simulink model "Part_3_Simulink_With_All_Scopes_Simplified_Blocks"  (R2016a)
settings: Solver=VariableStepAuto  StartTime=0.0  StopTime=12  RelTol=1e-3
values from neighbouring files (symbols this model uses):
  Alpha = 1    [Parameters_And_Plot.m]    (also in Part5_Specified_Destinations.m)
  K12 = K(1,2)    [Parameters_And_Plot.m]    (also in Part5_Specified_Destinations.m)
  K13 = K(1,3)    [Parameters_And_Plot.m]    (also in Part5_Specified_Destinations.m)
  K14 = K(1,4)    [Parameters_And_Plot.m]    (also in Part5_Specified_Destinations.m)
  K15 = K(1,5)    [Parameters_And_Plot.m]    (also in Part5_Specified_Destinations.m)
  K21 = K(2,1)    [Parameters_And_Plot.m]    (also in Part5_Specified_Destinations.m)
  K23 = K(2,1)    [Parameters_And_Plot.m]    (also in Part5_Specified_Destinations.m)
  K24 = K(2,1)    [Parameters_And_Plot.m]    (also in Part5_Specified_Destinations.m)
  K25 = K(2,1)    [Parameters_And_Plot.m]    (also in Part5_Specified_Destinations.m)
  K31 = K(3,1)    [Parameters_And_Plot.m]    (also in Part5_Specified_Destinations.m)
  K32 = K(3,2)    [Parameters_And_Plot.m]    (also in Part5_Specified_Destinations.m)
  K34 = K(3,4)    [Parameters_And_Plot.m]    (also in Part5_Specified_Destinations.m)
  K35 = K(3,5)    [Parameters_And_Plot.m]    (also in Part5_Specified_Destinations.m)
  K41 = K(4,1)    [Parameters_And_Plot.m]    (also in Part5_Specified_Destinations.m)
  K42 = K(4,2)    [Parameters_And_Plot.m]    (also in Part5_Specified_Destinations.m)
  K43 = K(4,3)    [Parameters_And_Plot.m]    (also in Part5_Specified_Destinations.m)
  K45 = K(4,5)    [Parameters_And_Plot.m]    (also in Part5_Specified_Destinations.m)
  K51 = K(5,1)    [Parameters_And_Plot.m]    (also in Part5_Specified_Destinations.m)
  K52 = K(5,2)    [Parameters_And_Plot.m]    (also in Part5_Specified_Destinations.m)
  K53 = K(5,3)    [Parameters_And_Plot.m]    (also in Part5_Specified_Destinations.m)
  K54 = K(5,4)    [Parameters_And_Plot.m]    (also in Part5_Specified_Destinations.m)
  L = 1    [Parameters_And_Plot.m]    (also in Part5_Specified_Destinations.m)
  x1_0 = r1_0(1)    [Parameters_And_Plot.m]    (also in Part5_Specified_Destinations.m)
  x1d = r1d(1)    [Parameters_And_Plot.m]    (also in Part5_Specified_Destinations.m)
  x2_0 = r2_0(1)    [Parameters_And_Plot.m]    (also in Part5_Specified_Destinations.m)
  x2d = r2d(1)    [Parameters_And_Plot.m]    (also in Part5_Specified_Destinations.m)
  x3_0 = r3_0(1)    [Parameters_And_Plot.m]    (also in Part5_Specified_Destinations.m)
  x3d = r3d(1)    [Parameters_And_Plot.m]    (also in Part5_Specified_Destinations.m)
  x4_0 = r4_0(1)    [Parameters_And_Plot.m]    (also in Part5_Specified_Destinations.m)
  x4d = r4d(1)    [Parameters_And_Plot.m]    (also in Part5_Specified_Destinations.m)
  x5_0 = r5_0(1)    [Parameters_And_Plot.m]    (also in Part5_Specified_Destinations.m)
  x5d = r5d(1)    [Parameters_And_Plot.m]    (also in Part5_Specified_Destinations.m)
  y1_0 = r1_0(2)    [Parameters_And_Plot.m]    (also in Part5_Specified_Destinations.m)
  y1d = r1d(2)    [Parameters_And_Plot.m]    (also in Part5_Specified_Destinations.m)
  y2_0 = r2_0(2)    [Parameters_And_Plot.m]    (also in Part5_Specified_Destinations.m)
  y2d = r2d(2)    [Parameters_And_Plot.m]    (also in Part5_Specified_Destinations.m)
  y3_0 = r3_0(2)    [Parameters_And_Plot.m]    (also in Part5_Specified_Destinations.m)
  y3d = r3d(2)    [Parameters_And_Plot.m]    (also in Part5_Specified_Destinations.m)
  y4_0 = r4_0(2)    [Parameters_And_Plot.m]    (also in Part5_Specified_Destinations.m)
  y4d = r4d(2)    [Parameters_And_Plot.m]    (also in Part5_Specified_Destinations.m)
  y5_0 = r5_0(2)    [Parameters_And_Plot.m]    (also in Part5_Specified_Destinations.m)
  y5d = r5d(2)    [Parameters_And_Plot.m]    (also in Part5_Specified_Destinations.m)
settings Model: Creator=Mohammad Hammoud  LastModifiedBy=Mohammad Hammoud

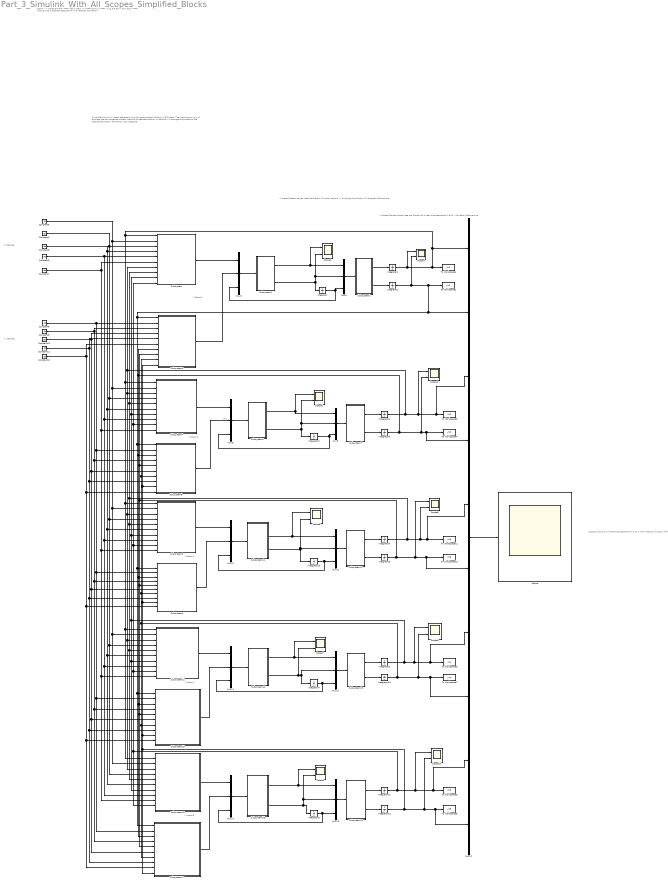
== system Part_3_Simulink_With_All_Scopes_Simplified_Blocks ==
  note: < Robot 1
  note: Yi desired
  note: Xi desired
  note: Scope to show all Linear Displacements
      | Xi and Yi of All Robots, function of Time
  note: In these Scopes we can see the Graphs of Linear
      | displacements Xi and Yi for each Robot alone
  note: In these Scopes we can see the Graphs of Linear Velocity Vi and Angular Velocity Wi for each Robot alone
  note: Part 3: " I mplement the controlled system in Matlab/Simulink "
      | Driving 5 Robots from their Initial Positions to a Desired destination
      | (with Desired Formation)
  note: Simplified Simulink Model representing a Consensus-based Control of 5 Robots,
      | The used control Law Ui, ensures the convergence of each robot to its desired position
      | In addition, it arranges the shape of the Desired Formation (Formation Convergence)
  note: Uy2
  note: < Robot 2
  note: < Robot 3
  note: < Robot 4
  note: < Robot 5
  Constant10 : Constant  Value=y3d
  Constant11 : Constant  Value=y4d
  Constant12 : Constant  Value=y5d
  Constant3 : Constant  Value=x1d
  Constant4 : Constant  Value=x2d
  Constant5 : Constant  Value=x3d
  Constant6 : Constant  Value=x4d
  Constant7 : Constant  Value=x5d
  Constant8 : Constant  Value=y1d
  Constant9 : Constant  Value=y2d
  Integrator{,1,4,6,10} (5 alike) : Integrator
  "Integrator1 " : Integrator  InitialCondition=x1_0
  "Integrator10 " : Integrator  InitialCondition=y4_0
  "Integrator11 " : Integrator  InitialCondition=x5_0
  "Integrator12 " : Integrator  InitialCondition=y5_0
  Integrator2 : Integrator  InitialCondition=y1_0
  Integrator3 : Integrator  InitialCondition=y2_0
  "Integrator4 " : Integrator  InitialCondition=x2_0
  "Integrator5 " : Integrator  InitialCondition=x3_0
  "Integrator8 " : Integrator  InitialCondition=y3_0
  "Integrator9 " : Integrator  InitialCondition=x4_0
  Mux{5..6,8..9,11..12,14..15,21..22} (10 alike) : Mux  Inputs=3
  Mux17 : Mux  Inputs=10
  Scope : Scope
  Scope{1..10} (10 alike) : Scope  NumInputPorts=2
  Subsystem : Subsystem
  Subsystem1 : Subsystem
  Subsystem10 : Subsystem
  Subsystem11 : Subsystem
  Subsystem12 : Subsystem
  Subsystem13 : Subsystem
  Subsystem14 : Subsystem
  Subsystem15 : Subsystem
  Subsystem16 : Subsystem
  Subsystem17 : Subsystem
  Subsystem18 : Subsystem
  Subsystem19 : Subsystem
  Subsystem2 : Subsystem
  Subsystem3 : Subsystem
  Subsystem4 : Subsystem
  Subsystem5 : Subsystem
  Subsystem6 : Subsystem
  Subsystem7 : Subsystem
  Subsystem8 : Subsystem
  Subsystem9 : Subsystem
  To Workspace1 : ToWorkspace  VariableName=xh1  SampleTime=-1
  To Workspace11 : ToWorkspace  VariableName=xh3  SampleTime=-1
  To Workspace12 : ToWorkspace  VariableName=yh3  SampleTime=-1
  To Workspace2 : ToWorkspace  VariableName=yh1  SampleTime=-1
  To Workspace3 : ToWorkspace  VariableName=xh2  SampleTime=-1
  To Workspace4 : ToWorkspace  VariableName=yh2  SampleTime=-1
  To Workspace5 : ToWorkspace  VariableName=xh5  SampleTime=-1
  To Workspace6 : ToWorkspace  VariableName=xh4  SampleTime=-1
  To Workspace7 : ToWorkspace  VariableName=yh4  SampleTime=-1
  To Workspace8 : ToWorkspace  VariableName=yh5  SampleTime=-1
  wires:
  Constant3/1 -> Subsystem16/2(In2), Subsystem12/2(In2), Subsystem8/2(In2), Subsystem4/2(In2), Subsystem/2(In2)  "x1d"
  Constant4/1 -> Subsystem16/4(In4), Subsystem12/4(In4), Subsystem8/4(In4), Subsystem4/4(In4), Subsystem/3(In3)  "x2d"
  Constant5/1 -> Subsystem16/6(In6), Subsystem12/6(In6), Subsystem8/6(In6), Subsystem4/6(In6), Subsystem/4(In4)  "x3d"
  Constant6/1 -> Subsystem16/8(In8), Subsystem12/8(In8), Subsystem8/8(In8), Subsystem4/8(In8), Subsystem/5(In5)  "x4d"
  Constant7/1 -> Subsystem16/9(In9), Subsystem12/10(In10), Subsystem8/10(In10), Subsystem4/10(In10), Subsystem/6(In6)  "x5d"
  Constant8/1 -> Subsystem17/2(In2), Subsystem13/2(In2), Subsystem9/2(In2), Subsystem5/2(In2), Subsystem3/2(In2)  "y1d"
  Constant9/1 -> Subsystem17/4(In4), Subsystem13/4(In4), Subsystem9/4(In4), Subsystem5/4(In4), Subsystem3/3(In3)  "y2d"
  Constant10/1 -> Subsystem3/4(In4), Subsystem17/6(In6), Subsystem13/6(In6), Subsystem9/6(In6), Subsystem5/6(In6)  "y3d"
  Constant11/1 -> Subsystem3/5(In5), Subsystem17/8(In8), Subsystem13/8(In8), Subsystem9/8(In8), Subsystem5/8(In8)  "y4d"
  Constant12/1 -> Subsystem3/6(In6), Subsystem17/9(In9), Subsystem13/10(In10), Subsystem9/10(In10), Subsystem5/10(In10)  "y5d"
  Integrator/1 -> Mux6/3, Mux5/3  "Theta 1"
  "Integrator1 "/1 -> Scope4/1, Subsystem/1(In1), Subsystem16/1(In1), Subsystem12/1(In1), Subsystem8/1(In1), Subsystem4/1(In1), Mux17/1, To Workspace1/1  "x1"
  Integrator2/1 -> To Workspace2/1, Subsystem3/1(In1), Subsystem17/1(In1), Subsystem13/1(In1), Subsystem9/1(In1), Subsystem5/1(In1), Mux17/2, Scope4/2  "y1"
  Integrator1/1 -> Mux8/3, Mux9/3  "Theta 2"
  "Integrator4 "/1 -> Subsystem/7(In7), Subsystem16/3(In3), Subsystem12/3(In3), Subsystem8/3(In3), Subsystem4/3(In3), Scope3/1, Mux17/3, To Workspace3/1  "x2"
  Integrator3/1 -> Subsystem3/7(In7), Subsystem5/3(In3), Subsystem13/3(In3), Subsystem17/3(In3), Subsystem9/3(In3), Scope3/2, To Workspace4/1, Mux17/4  "y2"
  Integrator10/1 -> Mux22/3, Mux21/3  "Theta 3"
  "Integrator5 "/1 -> Subsystem/8(In8), Subsystem4/5(In5), Subsystem16/5(In5), Subsystem12/5(In5), Subsystem8/5(In5), Scope6/2, Mux17/5, To Workspace11/1  "x3"
  "Integrator8 "/1 -> Subsystem3/8(In8), Subsystem5/5(In5), Subsystem17/5(In5), Subsystem13/5(In5), Subsystem9/5(In5), Scope6/1, To Workspace12/1, Mux17/6  "y3"
  Integrator4/1 -> Mux11/3, Mux12/3  "Theta 4"
  "Integrator9 "/1 -> To Workspace6/1, Mux17/7, Scope8/1, Subsystem16/7(In7), Subsystem12/7(In7), Subsystem/9(In9), Subsystem4/7(In7), Subsystem8/7(In7)  "x4"
  "Integrator10 "/1 -> To Workspace7/1, Mux17/8, Scope8/2, Subsystem3/9(In9), Subsystem5/7(In7), Subsystem9/7(In7), Subsystem17/7(In7), Subsystem13/7(In7)  "y4"
  Integrator6/1 -> Mux15/3, Mux14/3  "Theta 5"
  "Integrator11 "/1 -> To Workspace5/1, Mux17/9, Scope10/1, Subsystem/10(In10), Subsystem4/9(In9), Subsystem8/9(In9), Subsystem12/9(In9), Subsystem16/10(In10)  "x5"
  "Integrator12 "/1 -> To Workspace8/1, Mux17/10, Scope10/2, Subsystem17/10(In10), Subsystem3/10(In10), Subsystem5/9(In9), Subsystem9/9(In9), Subsystem13/9(In9)  "y5"
  Mux17/1 -> Scope/1
  Subsystem/1(Out1) -> Mux5/1  "Ux1"
  Subsystem1/2(Out2) -> Scope1/2, Mux6/2, Integrator/1  "W1"
  Subsystem1/1(Out1) -> Scope1/1, Mux6/1  "V1"
  Mux5/1 -> Subsystem1/1(In1)
  Mux6/1 -> Subsystem2/1(In1)
  Subsystem2/1(Out1) -> "Integrator1 "/1  "x1dot"
  Subsystem2/2(Out2) -> Integrator2/1  "y1dot"
  Subsystem3/1(Out1) -> Mux5/2  "Uy1"
  Subsystem4/1(Out1) -> Mux8/1  "Ux2"
  Subsystem5/1(Out1) -> Mux8/2
  Subsystem6/2(Out2) -> Integrator1/1, Scope2/2, Mux9/2  "W2"
  Subsystem6/1(Out1) -> Mux9/1, Scope2/1  "V2"
  Mux8/1 -> Subsystem6/1(In1)
  Mux9/1 -> Subsystem7/1(In1)
  Subsystem7/1(Out1) -> "Integrator4 "/1  "x2dot"
  Subsystem7/2(Out2) -> Integrator3/1  "y2dot"
  Subsystem8/1(Out1) -> Mux21/1  "Ux3"
  Subsystem9/1(Out1) -> Mux21/2  "Uy3"
  Subsystem10/1(Out1) -> Scope5/1, Mux22/1  "V3"
  Subsystem10/2(Out2) -> Integrator10/1, Scope5/2, Mux22/2  "W3"
  Mux21/1 -> Subsystem10/1(In1)
  Mux22/1 -> Subsystem11/1(In1)
  Subsystem11/1(Out1) -> "Integrator5 "/1  "x3dot"
  Subsystem11/2(Out2) -> "Integrator8 "/1  "y3dot"
  Subsystem12/1(Out1) -> Mux11/1  "Ux4"
  Subsystem13/1(Out1) -> Mux11/2  "Uy4"
  Subsystem14/1(Out1) -> Scope7/1, Mux12/1  "V4"
  Subsystem14/2(Out2) -> Scope7/2, Mux12/2, Integrator4/1  "W4"
  Mux11/1 -> Subsystem14/1(In1)
  Mux12/1 -> Subsystem15/1(In1)
  Subsystem15/1(Out1) -> "Integrator9 "/1  "x4dot"
  Subsystem15/2(Out2) -> "Integrator10 "/1  "y4dot"
  Subsystem16/1(Out1) -> Mux14/1  "Ux5"
  Subsystem17/1(Out1) -> Mux14/2  "Uy5"
  Subsystem18/1(Out1) -> Scope9/1, Mux15/1  "V5"
  Subsystem18/2(Out2) -> Integrator6/1, Scope9/2, Mux15/2  "W5"
  Mux14/1 -> Subsystem18/1(In1)
  Mux15/1 -> Subsystem19/1(In1)
  Subsystem19/1(Out1) -> "Integrator11 "/1  "x5dot"
  Subsystem19/2(Out2) -> "Integrator12 "/1  "y5dot"

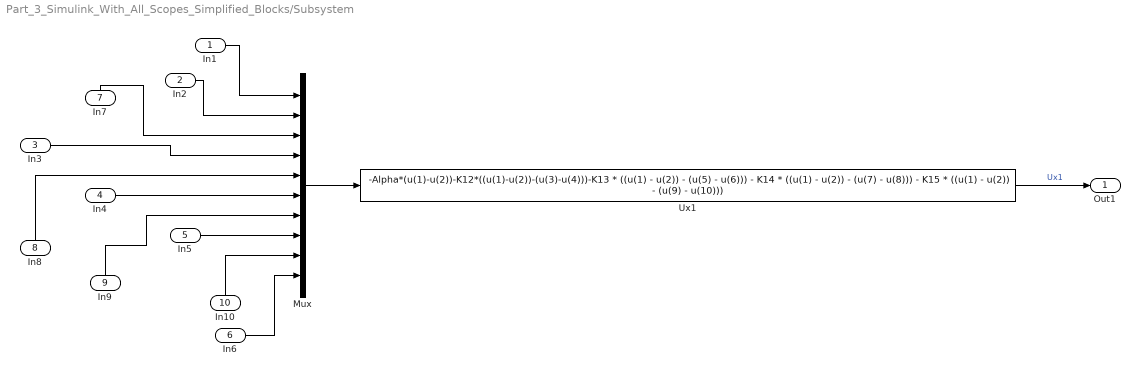
== system Part_3_Simulink_With_All_Scopes_Simplified_Blocks/Subsystem ==
  In1 : Inport
  In2 : Inport  Port=2
  In3 : Inport  Port=3
  In4 : Inport  Port=4
  In5 : Inport  Port=5
  In6 : Inport  Port=6
  In7 : Inport  Port=7
  In8 : Inport  Port=8
  In9 : Inport  Port=9
  In10 : Inport  Port=10
  Mux : Mux  Inputs=10
  Ux1 : Fcn  Expr=-Alpha*(u(1)-u(2))-K12*((u(1)-u(2))-(u(3)-u(4)))-K13 * ((u(1) - u(2)) - (u(5) - u(6))) - K14 * ((u(1) - u(2)) - (u(7) - u(8))) - K15 * ((u(1) - u(2)) - (u(9) - u(10)))
  Out1 : Outport
  wires:
  In9/1 -> Mux/7
  In2/1 -> Mux/2
  In3/1 -> Mux/4
  In4/1 -> Mux/6
  In1/1 -> Mux/1
  In6/1 -> Mux/10
  In5/1 -> Mux/8
  In10/1 -> Mux/9
  In8/1 -> Mux/5
  In7/1 -> Mux/3
  Mux/1 -> Ux1/1
  Ux1/1 -> Out1/1  "Ux1"

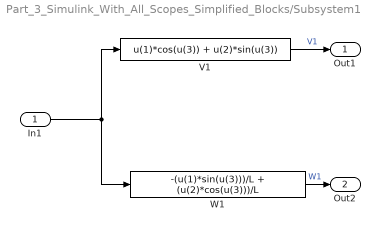
== system Part_3_Simulink_With_All_Scopes_Simplified_Blocks/Subsystem1 ==
  In1 : Inport
  V1 : Fcn  Expr=u(1)*cos(u(3)) + u(2)*sin(u(3))
  W1 : Fcn  Expr=-(u(1)*sin(u(3)))/L + (u(2)*cos(u(3)))/L
  Out1 : Outport
  Out2 : Outport  Port=2
  wires:
  In1/1 -> V1/1, W1/1
  V1/1 -> Out1/1  "V1"
  W1/1 -> Out2/1  "W1"

== system Part_3_Simulink_With_All_Scopes_Simplified_Blocks/Subsystem10 ==
  In1 : Inport
  V3 : Fcn  Expr=u(1)*cos(u(3)) + u(2)*sin(u(3))
  W3 : Fcn  Expr=-(u(1)*sin(u(3)))/L + (u(2)*cos(u(3)))/L
  Out1 : Outport
  Out2 : Outport  Port=2
  wires:
  W3/1 -> Out2/1  "W3"
  V3/1 -> Out1/1  "V3"
  In1/1 -> V3/1, W3/1

== system Part_3_Simulink_With_All_Scopes_Simplified_Blocks/Subsystem11 ==
  In1 : Inport
  Xhdot 3 : Fcn  Expr=u(1)*cos(u(3)) - L*u(2)*sin(u(3))
  Yhdot 3 : Fcn  Expr=u(1)*sin(u(3)) + L*u(2)*cos(u(3))
  Out1 : Outport
  Out2 : Outport  Port=2
  wires:
  In1/1 -> Yhdot 3/1, Xhdot 3/1
  Yhdot 3/1 -> Out2/1
  Xhdot 3/1 -> Out1/1

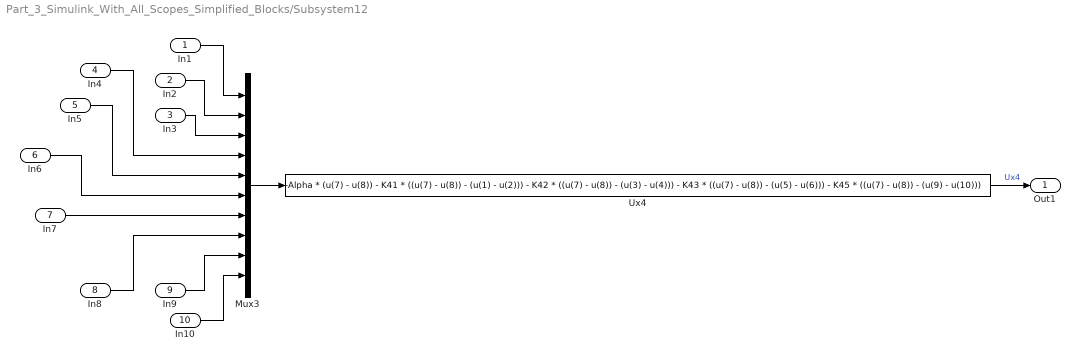
== system Part_3_Simulink_With_All_Scopes_Simplified_Blocks/Subsystem12 ==
  In1 : Inport
  In2 : Inport  Port=2
  In3 : Inport  Port=3
  In4 : Inport  Port=4
  In5 : Inport  Port=5
  In6 : Inport  Port=6
  In7 : Inport  Port=7
  In8 : Inport  Port=8
  In9 : Inport  Port=9
  In10 : Inport  Port=10
  Mux3 : Mux  Inputs=10
  Ux4 : Fcn  Expr=-Alpha * (u(7) - u(8)) - K41 * ((u(7) - u(8)) - (u(1) - u(2))) - K42 * ((u(7) - u(8)) - (u(3) - u(4))) - K43 * ((u(7) - u(8)) - (u(5) - u(6))) - K45 * ((u(7) - u(8)) - (u(9) - u(10)))
  Out1 : Outport
  wires:
  In9/1 -> Mux3/9
  In3/1 -> Mux3/3
  In7/1 -> Mux3/7
  In4/1 -> Mux3/4
  In10/1 -> Mux3/10
  In1/1 -> Mux3/1
  In2/1 -> Mux3/2
  In5/1 -> Mux3/5
  In6/1 -> Mux3/6
  In8/1 -> Mux3/8
  Mux3/1 -> Ux4/1
  Ux4/1 -> Out1/1  "Ux4"

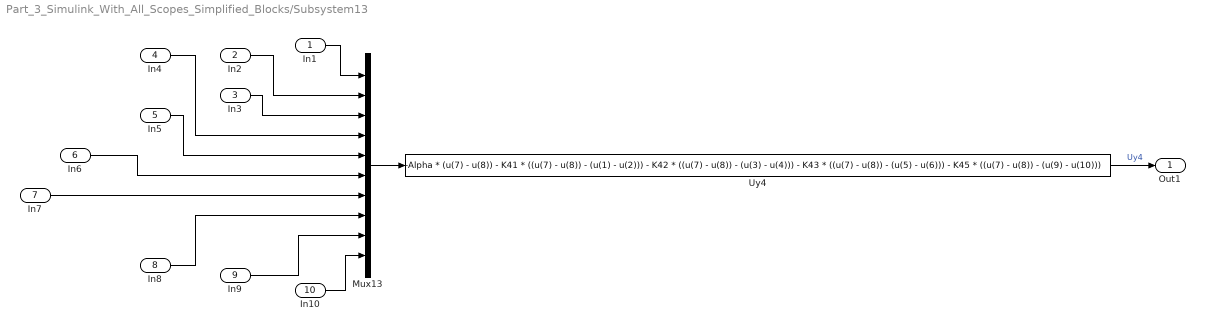
== system Part_3_Simulink_With_All_Scopes_Simplified_Blocks/Subsystem13 ==
  In1 : Inport
  In2 : Inport  Port=2
  In3 : Inport  Port=3
  In4 : Inport  Port=4
  In5 : Inport  Port=5
  In6 : Inport  Port=6
  In7 : Inport  Port=7
  In8 : Inport  Port=8
  In9 : Inport  Port=9
  In10 : Inport  Port=10
  Mux13 : Mux  Inputs=10
  Uy4 : Fcn  Expr=-Alpha * (u(7) - u(8)) - K41 * ((u(7) - u(8)) - (u(1) - u(2))) - K42 * ((u(7) - u(8)) - (u(3) - u(4))) - K43 * ((u(7) - u(8)) - (u(5) - u(6))) - K45 * ((u(7) - u(8)) - (u(9) - u(10)))
  Out1 : Outport
  wires:
  In5/1 -> Mux13/5
  In1/1 -> Mux13/1
  In7/1 -> Mux13/7
  In6/1 -> Mux13/6
  In9/1 -> Mux13/9
  In4/1 -> Mux13/4
  In8/1 -> Mux13/8
  In2/1 -> Mux13/2
  In10/1 -> Mux13/10
  In3/1 -> Mux13/3
  Mux13/1 -> Uy4/1
  Uy4/1 -> Out1/1  "Uy4"

== system Part_3_Simulink_With_All_Scopes_Simplified_Blocks/Subsystem14 ==
  In1 : Inport
  V4 : Fcn  Expr=u(1)*cos(u(3)) + u(2)*sin(u(3))
  W4 : Fcn  Expr=-(u(1)*sin(u(3)))/L + (u(2)*cos(u(3)))/L
  Out1 : Outport
  Out2 : Outport  Port=2
  wires:
  In1/1 -> W4/1, V4/1
  W4/1 -> Out2/1  "W4"
  V4/1 -> Out1/1  "V4"

== system Part_3_Simulink_With_All_Scopes_Simplified_Blocks/Subsystem15 ==
  In1 : Inport
  Xhdot 4 : Fcn  Expr=u(1)*cos(u(3)) - L*u(2)*sin(u(3))
  Yhdot 4 : Fcn  Expr=u(1)*sin(u(3)) + L*u(2)*cos(u(3))
  Out1 : Outport
  Out2 : Outport  Port=2
  wires:
  Xhdot 4/1 -> Out1/1
  In1/1 -> Yhdot 4/1, Xhdot 4/1
  Yhdot 4/1 -> Out2/1

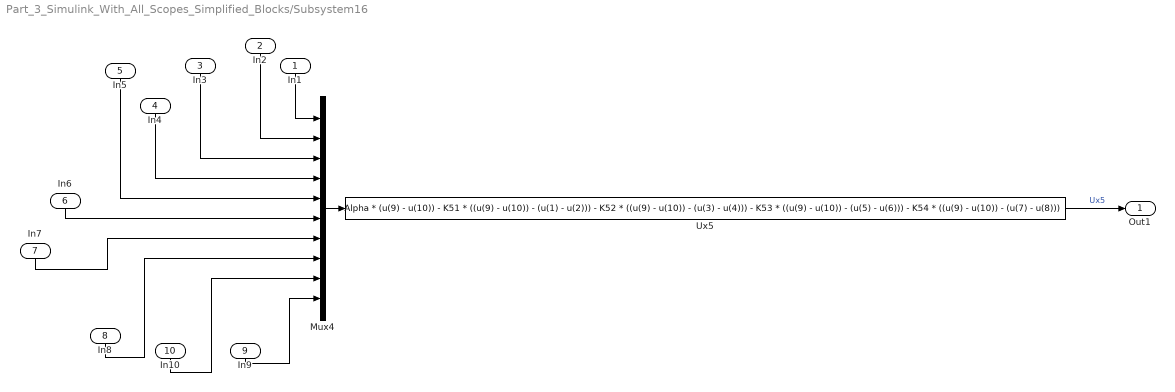
== system Part_3_Simulink_With_All_Scopes_Simplified_Blocks/Subsystem16 ==
  In1 : Inport
  In2 : Inport  Port=2
  In3 : Inport  Port=3
  In4 : Inport  Port=4
  In5 : Inport  Port=5
  In6 : Inport  Port=6
  In7 : Inport  Port=7
  In8 : Inport  Port=8
  In9 : Inport  Port=9
  In10 : Inport  Port=10
  Mux4 : Mux  Inputs=10
  Ux5 : Fcn  Expr=-Alpha * (u(9) - u(10)) - K51 * ((u(9) - u(10)) - (u(1) - u(2))) - K52 * ((u(9) - u(10)) - (u(3) - u(4))) - K53 * ((u(9) - u(10)) - (u(5) - u(6))) - K54 * ((u(9) - u(10)) - (u(7) - u(8)))
  Out1 : Outport
  wires:
  Mux4/1 -> Ux5/1
  Ux5/1 -> Out1/1  "Ux5"
  In6/1 -> Mux4/6
  In10/1 -> Mux4/9
  In9/1 -> Mux4/10
  In4/1 -> Mux4/4
  In8/1 -> Mux4/8
  In1/1 -> Mux4/1
  In2/1 -> Mux4/2
  In3/1 -> Mux4/3
  In7/1 -> Mux4/7
  In5/1 -> Mux4/5

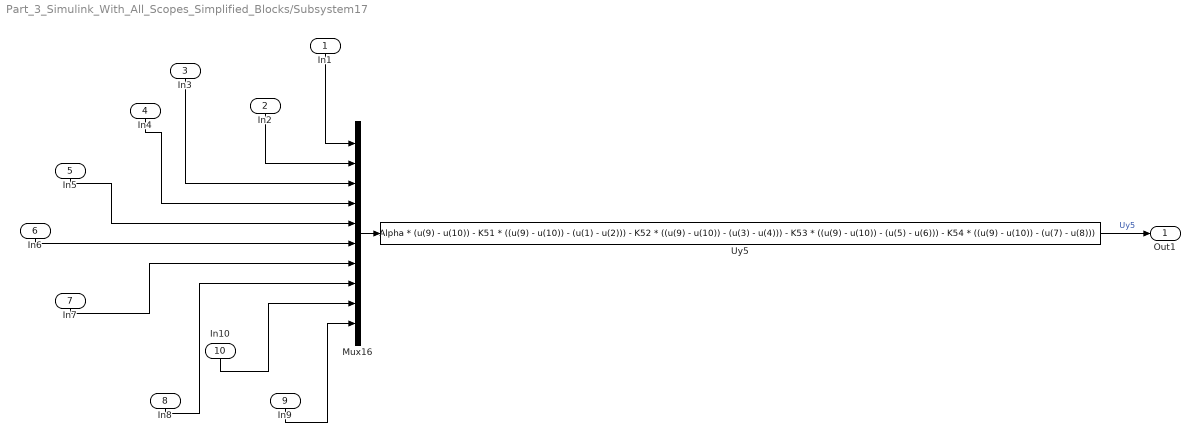
== system Part_3_Simulink_With_All_Scopes_Simplified_Blocks/Subsystem17 ==
  In1 : Inport
  In2 : Inport  Port=2
  In3 : Inport  Port=3
  In4 : Inport  Port=4
  In5 : Inport  Port=5
  In6 : Inport  Port=6
  In7 : Inport  Port=7
  In8 : Inport  Port=8
  In9 : Inport  Port=9
  In10 : Inport  Port=10
  Mux16 : Mux  Inputs=10
  Uy5 : Fcn  Expr=-Alpha * (u(9) - u(10)) - K51 * ((u(9) - u(10)) - (u(1) - u(2))) - K52 * ((u(9) - u(10)) - (u(3) - u(4))) - K53 * ((u(9) - u(10)) - (u(5) - u(6))) - K54 * ((u(9) - u(10)) - (u(7) - u(8)))
  Out1 : Outport
  wires:
  In10/1 -> Mux16/9
  In8/1 -> Mux16/8
  In4/1 -> Mux16/4
  In5/1 -> Mux16/5
  In2/1 -> Mux16/2
  In1/1 -> Mux16/1
  In6/1 -> Mux16/6
  In7/1 -> Mux16/7
  In3/1 -> Mux16/3
  In9/1 -> Mux16/10
  Mux16/1 -> Uy5/1
  Uy5/1 -> Out1/1  "Uy5"

== system Part_3_Simulink_With_All_Scopes_Simplified_Blocks/Subsystem18 ==
  In1 : Inport
  V5 : Fcn  Expr=u(1)*cos(u(3)) + u(2)*sin(u(3))
  W5 : Fcn  Expr=-(u(1)*sin(u(3)))/L + (u(2)*cos(u(3)))/L
  Out1 : Outport
  Out2 : Outport  Port=2
  wires:
  W5/1 -> Out2/1  "W5"
  In1/1 -> W5/1, V5/1
  V5/1 -> Out1/1  "V5"

== system Part_3_Simulink_With_All_Scopes_Simplified_Blocks/Subsystem19 ==
  In1 : Inport
  Xhdot 5 : Fcn  Expr=u(1)*cos(u(3)) - L*u(2)*sin(u(3))
  Yhdot 5 : Fcn  Expr=u(1)*sin(u(3)) + L*u(2)*cos(u(3))
  Out1 : Outport
  Out2 : Outport  Port=2
  wires:
  In1/1 -> Yhdot 5/1, Xhdot 5/1
  Yhdot 5/1 -> Out2/1
  Xhdot 5/1 -> Out1/1

== system Part_3_Simulink_With_All_Scopes_Simplified_Blocks/Subsystem2 ==
  In1 : Inport
  Xhdot 1 : Fcn  Expr=u(1)*cos(u(3)) - L*u(2)*sin(u(3))
  Yhdot 1 : Fcn  Expr=u(1)*sin(u(3)) + L*u(2)*cos(u(3))
  Out1 : Outport
  Out2 : Outport  Port=2
  wires:
  In1/1 -> Xhdot 1/1, Yhdot 1/1
  Yhdot 1/1 -> Out2/1
  Xhdot 1/1 -> Out1/1

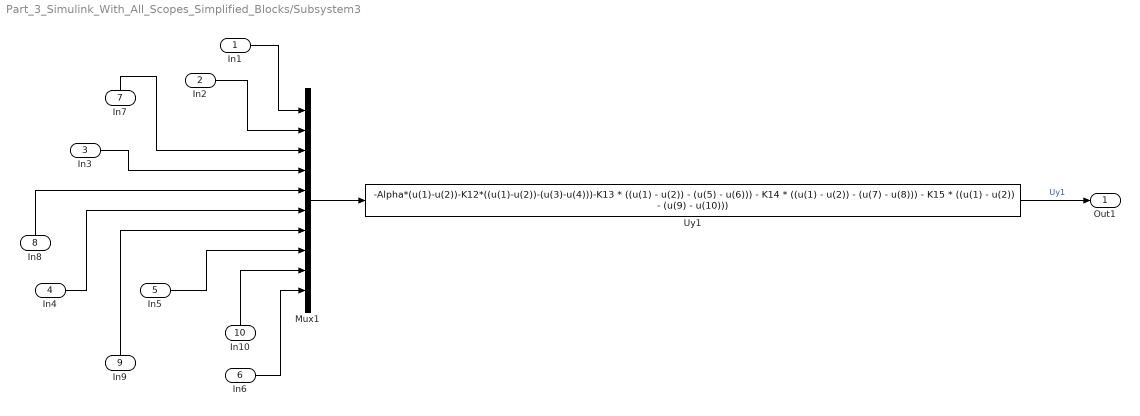
== system Part_3_Simulink_With_All_Scopes_Simplified_Blocks/Subsystem3 ==
  In1 : Inport
  In2 : Inport  Port=2
  In3 : Inport  Port=3
  In4 : Inport  Port=4
  In5 : Inport  Port=5
  In6 : Inport  Port=6
  In7 : Inport  Port=7
  In8 : Inport  Port=8
  In9 : Inport  Port=9
  In10 : Inport  Port=10
  Mux1 : Mux  Inputs=10
  Uy1 : Fcn  Expr=-Alpha*(u(1)-u(2))-K12*((u(1)-u(2))-(u(3)-u(4)))-K13 * ((u(1) - u(2)) - (u(5) - u(6))) - K14 * ((u(1) - u(2)) - (u(7) - u(8))) - K15 * ((u(1) - u(2)) - (u(9) - u(10)))
  Out1 : Outport
  wires:
  In10/1 -> Mux1/9
  In9/1 -> Mux1/7
  In8/1 -> Mux1/5
  In5/1 -> Mux1/8
  In7/1 -> Mux1/3
  In1/1 -> Mux1/1
  In3/1 -> Mux1/4
  In4/1 -> Mux1/6
  In6/1 -> Mux1/10
  In2/1 -> Mux1/2
  Mux1/1 -> Uy1/1
  Uy1/1 -> Out1/1  "Uy1"

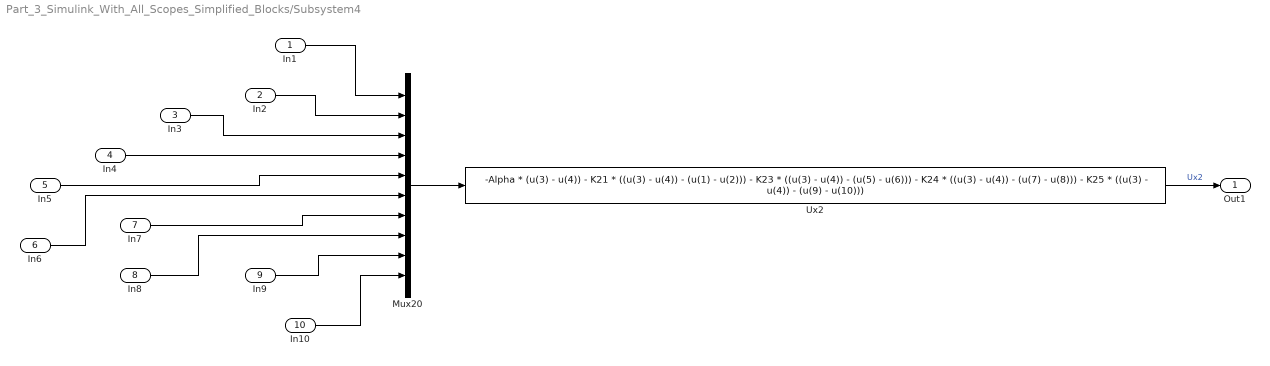
== system Part_3_Simulink_With_All_Scopes_Simplified_Blocks/Subsystem4 ==
  In1 : Inport
  In2 : Inport  Port=2
  In3 : Inport  Port=3
  In4 : Inport  Port=4
  In5 : Inport  Port=5
  In6 : Inport  Port=6
  In7 : Inport  Port=7
  In8 : Inport  Port=8
  In9 : Inport  Port=9
  In10 : Inport  Port=10
  Mux20 : Mux  Inputs=10
  Ux2 : Fcn  Expr=-Alpha * (u(3) - u(4)) - K21 * ((u(3) - u(4)) - (u(1) - u(2))) - K23 * ((u(3) - u(4)) - (u(5) - u(6))) - K24 * ((u(3) - u(4)) - (u(7) - u(8))) - K25 * ((u(3) - u(4)) - (u(9) - u(10)))
  Out1 : Outport
  wires:
  In5/1 -> Mux20/5
  In7/1 -> Mux20/7
  In8/1 -> Mux20/8
  In10/1 -> Mux20/10
  In6/1 -> Mux20/6
  In4/1 -> Mux20/4
  In1/1 -> Mux20/1
  In3/1 -> Mux20/3
  In9/1 -> Mux20/9
  In2/1 -> Mux20/2
  Mux20/1 -> Ux2/1
  Ux2/1 -> Out1/1  "Ux2"

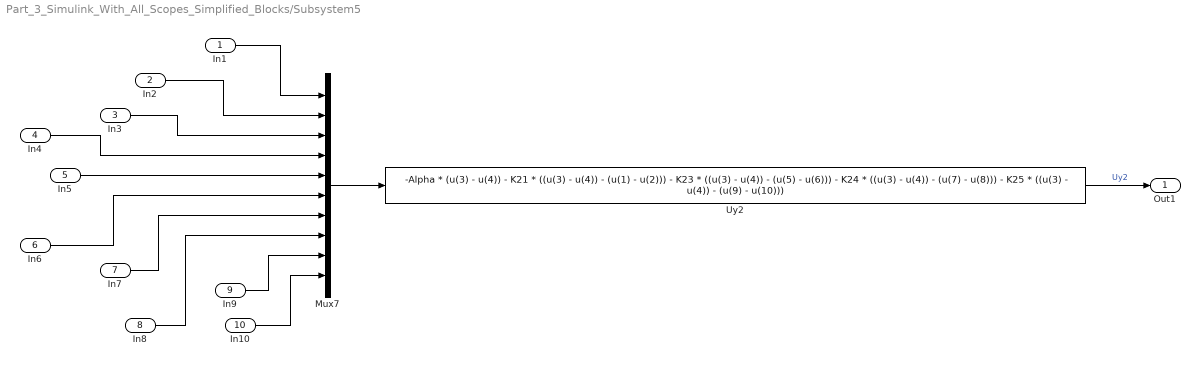
== system Part_3_Simulink_With_All_Scopes_Simplified_Blocks/Subsystem5 ==
  In1 : Inport
  In2 : Inport  Port=2
  In3 : Inport  Port=3
  In4 : Inport  Port=4
  In5 : Inport  Port=5
  In6 : Inport  Port=6
  In7 : Inport  Port=7
  In8 : Inport  Port=8
  In9 : Inport  Port=9
  In10 : Inport  Port=10
  Mux7 : Mux  Inputs=10
  Uy2 : Fcn  Expr=-Alpha * (u(3) - u(4)) - K21 * ((u(3) - u(4)) - (u(1) - u(2))) - K23 * ((u(3) - u(4)) - (u(5) - u(6))) - K24 * ((u(3) - u(4)) - (u(7) - u(8))) - K25 * ((u(3) - u(4)) - (u(9) - u(10)))
  Out1 : Outport
  wires:
  In7/1 -> Mux7/7
  In5/1 -> Mux7/5
  In6/1 -> Mux7/6
  In2/1 -> Mux7/2
  In3/1 -> Mux7/3
  In8/1 -> Mux7/8
  In9/1 -> Mux7/9
  In1/1 -> Mux7/1
  In10/1 -> Mux7/10
  In4/1 -> Mux7/4
  Mux7/1 -> Uy2/1
  Uy2/1 -> Out1/1  "Uy2"

== system Part_3_Simulink_With_All_Scopes_Simplified_Blocks/Subsystem6 ==
  In1 : Inport
  V2 : Fcn  Expr=u(1)*cos(u(3)) + u(2)*sin(u(3))
  W2 : Fcn  Expr=-(u(1)*sin(u(3)))/L + (u(2)*cos(u(3)))/L
  Out1 : Outport
  Out2 : Outport  Port=2
  wires:
  In1/1 -> W2/1, V2/1
  W2/1 -> Out2/1  "W2"
  V2/1 -> Out1/1  "V2"

== system Part_3_Simulink_With_All_Scopes_Simplified_Blocks/Subsystem7 ==
  In1 : Inport
  Xhdot 2 : Fcn  Expr=u(1)*cos(u(3)) - L*u(2)*sin(u(3))
  Yhdot 2 : Fcn  Expr=u(1)*sin(u(3)) + L*u(2)*cos(u(3))
  Out1 : Outport
  Out2 : Outport  Port=2
  wires:
  In1/1 -> Yhdot 2/1, Xhdot 2/1
  Yhdot 2/1 -> Out2/1
  Xhdot 2/1 -> Out1/1

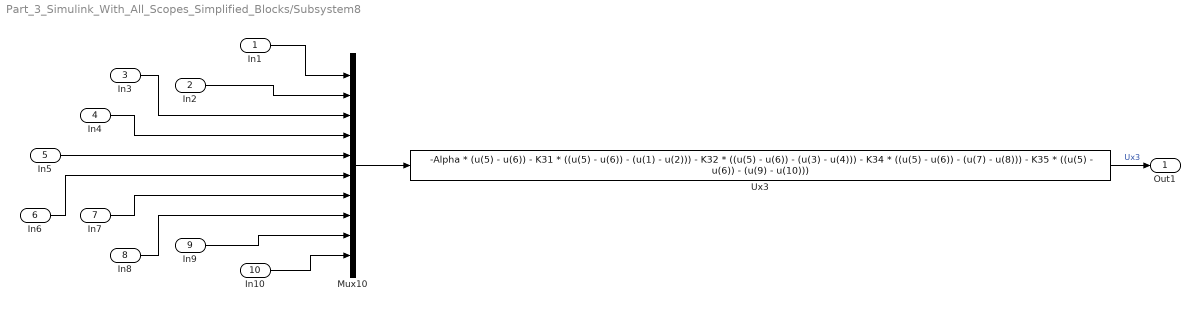
== system Part_3_Simulink_With_All_Scopes_Simplified_Blocks/Subsystem8 ==
  In1 : Inport
  In2 : Inport  Port=2
  In3 : Inport  Port=3
  In4 : Inport  Port=4
  In5 : Inport  Port=5
  In6 : Inport  Port=6
  In7 : Inport  Port=7
  In8 : Inport  Port=8
  In9 : Inport  Port=9
  In10 : Inport  Port=10
  Mux10 : Mux  Inputs=10
  Ux3 : Fcn  Expr=-Alpha * (u(5) - u(6)) - K31 * ((u(5) - u(6)) - (u(1) - u(2))) - K32 * ((u(5) - u(6)) - (u(3) - u(4))) - K34 * ((u(5) - u(6)) - (u(7) - u(8))) - K35 * ((u(5) - u(6)) - (u(9) - u(10)))
  Out1 : Outport
  wires:
  In9/1 -> Mux10/9
  In7/1 -> Mux10/7
  In2/1 -> Mux10/2
  In5/1 -> Mux10/5
  In3/1 -> Mux10/3
  In4/1 -> Mux10/4
  In8/1 -> Mux10/8
  In10/1 -> Mux10/10
  In1/1 -> Mux10/1
  In6/1 -> Mux10/6
  Ux3/1 -> Out1/1  "Ux3"
  Mux10/1 -> Ux3/1

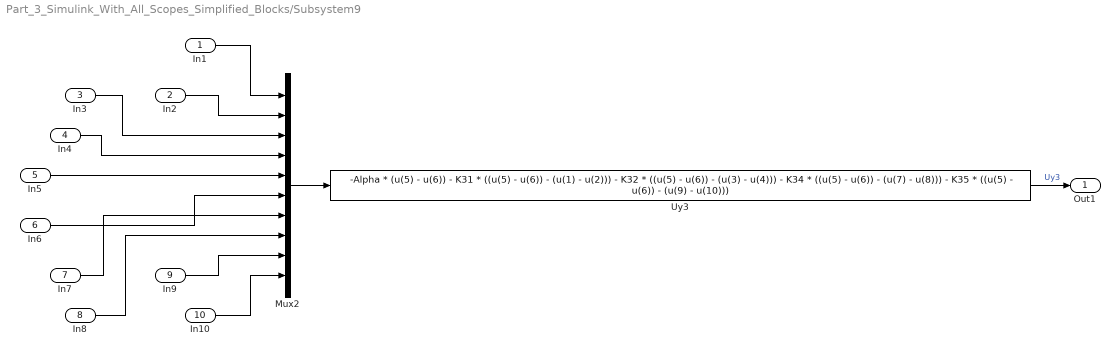
== system Part_3_Simulink_With_All_Scopes_Simplified_Blocks/Subsystem9 ==
  In1 : Inport
  In2 : Inport  Port=2
  In3 : Inport  Port=3
  In4 : Inport  Port=4
  In5 : Inport  Port=5
  In6 : Inport  Port=6
  In7 : Inport  Port=7
  In8 : Inport  Port=8
  In9 : Inport  Port=9
  In10 : Inport  Port=10
  Mux2 : Mux  Inputs=10
  Uy3 : Fcn  Expr=-Alpha * (u(5) - u(6)) - K31 * ((u(5) - u(6)) - (u(1) - u(2))) - K32 * ((u(5) - u(6)) - (u(3) - u(4))) - K34 * ((u(5) - u(6)) - (u(7) - u(8))) - K35 * ((u(5) - u(6)) - (u(9) - u(10)))
  Out1 : Outport
  wires:
  In3/1 -> Mux2/3
  In8/1 -> Mux2/8
  In4/1 -> Mux2/4
  In7/1 -> Mux2/7
  In5/1 -> Mux2/5
  In9/1 -> Mux2/9
  In1/1 -> Mux2/1
  In6/1 -> Mux2/6
  In10/1 -> Mux2/10
  In2/1 -> Mux2/2
  Mux2/1 -> Uy3/1
  Uy3/1 -> Out1/1  "Uy3"
